simulink model "DC_DC"  (R2021a)
settings: Solver=ode4  StartTime=0.0  StopTime=10.0  FixedStep=10e-6  RelTol=1e-3
libraries: spsSeriesRLCBranchLib x4, spsCurrentMeasurementLib x3, spsVoltageMeasurementLib x3, spsMeanLib x2, spsRMSLib x2, spsDiodeLib x1, spsFirstOrderFilterLib x1, spsIGBTDiodeLib x1, spsPermanentMagnetSynchronousMachineLib x1, simulink x1, spsThreePhaseVIMeasurementLib x1, spsUniversalBridgeLib x1
settings Model: Creator=Sourav Das  LastModifiedBy=Sourav Das

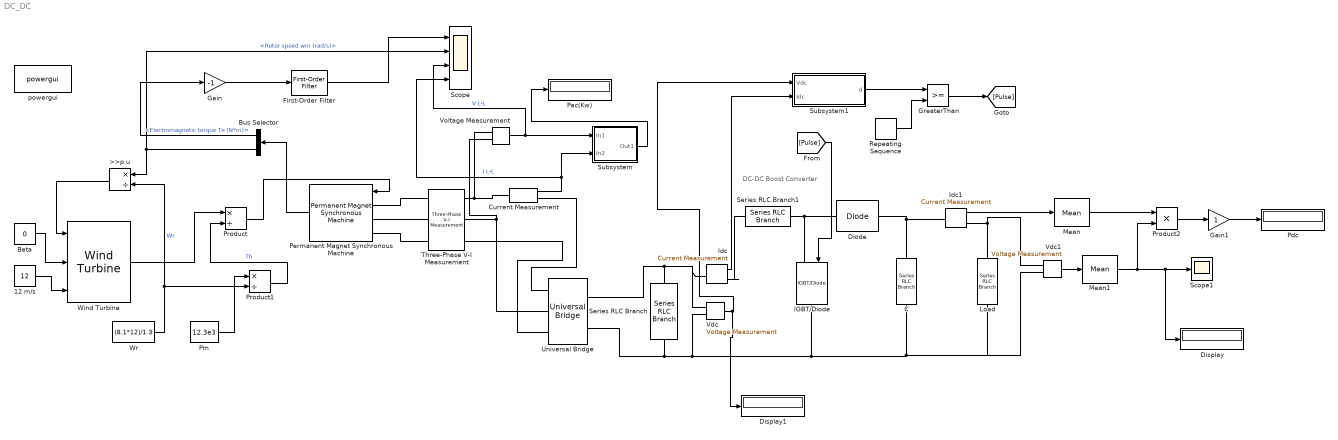
== system DC_DC ==
  note: DC-DC Boost Converter
  12 m/s : Constant  Value=12
  >>p.u : Product  Inputs=*/
  Beta : Constant  Value=0
  Bus Selector : BusSelector  OutputSignals=Electromagnetic torque Te (N*m),Rotor speed wm (rad/s)
  C : spsSeriesRLCBranchLib/Series RLC Branch  LConnTagsString=__new0  RConnTagsString=__new0  BranchType=RC  Resistance=0.005  Inductance=1e-3  SetiL0=off  InitialCurrent=0  Capacitance=6.6094e-04  Setx0=off  InitialVoltage=0  Measurements=None
  Current Measurement : spsCurrentMeasurementLib/Current Measurement  PhasorSimulation=off  OutputType=Complex  PSBequivalent=0
  Diode : spsDiodeLib/Diode  Ron=0.001  Lon=0  Vf=0.8  IC=0  UseSnubber=0  Rs=inf  Cs=inf  Measurements=off
  Display : Display
  Display1 : Display
  First-Order Filter : spsFirstOrderFilterLib/First-Order Filter  FilterType=Lowpass  Tc=10e-3  Ts=50e-6  Initialize=on  Vac_Init=[0, 0, 50]  Vdc_Init=0  PlotResponse=off  FreqRange="[0,  200,  1]"
  Gain : Gain  Gain=-1
  Gain1 : Gain
  GreaterThan : RelationalOperator  OutDataTypeStr=boolean  RndMeth=Simplest
  IGBT/Diode : spsIGBTDiodeLib/IGBT//Diode  Ron=1e-3  Rs=1e5  Cs=inf  Measurements=off
  Idc : spsCurrentMeasurementLib/Current Measurement  PhasorSimulation=off  OutputType=Complex  PSBequivalent=0
  Idc1 : spsCurrentMeasurementLib/Current Measurement  PhasorSimulation=off  OutputType=Complex  PSBequivalent=0
  Load : spsSeriesRLCBranchLib/Series RLC Branch  LConnTagsString=__new0  RConnTagsString=__new0  BranchType=R  Resistance=13.5  Inductance=1e-3  SetiL0=off  InitialCurrent=0  Capacitance=500e-6  Setx0=off  InitialVoltage=0  Measurements=None
  Mean : spsMeanLib/Mean  Freq=50  Vinit=0  Ts=50e-6
  Mean1 : spsMeanLib/Mean  Freq=50  Vinit=0  Ts=50e-6
  Pac(Kw) : Display
  Pdc : Display
  Permanent Magnet Synchronous Machine : spsPermanentMagnetSynchronousMachineLib/Permanent Magnet Synchronous Machine  NbPhases=3  FluxDistribution=Sinusoidal  RotorType=Salient-pole  MechanicalLoad=Torque Tm  PresetModel=No  ShowDetailedParameters=on  MeasurementBus=off  Resistance=0.0485  Inductance=8.5e-3  dqInductances=[0.395e-3,0.395e-3]  La=0.000395  MachineConstant=Flux linkage established by magnets (V.s)  Flux=0.1194  VoltageCst=86.6271  TorqueCst=0.7164  Flat=120  Mechanical=[0.0027 0.0004924 4 0]  PolePairs=4  InitialConditions=[0,0, 0,0]  InitialConditions5ph=[0 0 0 0 0 0]  RefAngle=90 degrees behind phase A axis (modified Park)  IterativeDiscreteModel=Trapezoidal non iterative  TsBlock=-1  TsPowergui=0
  Pm : Constant  Value=12.3e3
  Product : Product  Inputs=*/
  Product1 : Product  Inputs=*/
  Product2 : Product
  Repeating Sequence : simulink/Sources/Repeating Sequence  rep_seq_t=[0 1/20000]  rep_seq_y=[0 0.9]
  Scope : Scope  NumInputPorts=4
  Scope1 : Scope
  Series RLC Branch : spsSeriesRLCBranchLib/Series RLC Branch  LConnTagsString=__new0  RConnTagsString=__new0  BranchType=RC  Resistance=0.005  Inductance=1e-3  SetiL0=off  InitialCurrent=0  Capacitance=500e-6  Setx0=off  InitialVoltage=0  Measurements=None
  Series RLC Branch1 : spsSeriesRLCBranchLib/Series RLC Branch  LConnTagsString=__new0  RConnTagsString=__new0  BranchType=L  Resistance=0.005  Inductance=4.5573e-05  SetiL0=off  InitialCurrent=0  Capacitance=500e-6  Setx0=off  InitialVoltage=0  Measurements=None
  Subsystem : Subsystem
  Subsystem1 : Subsystem
  Three-Phase V-I Measurement : spsThreePhaseVIMeasurementLib/Three-Phase V-I Measurement  VoltageMeasurement=no  SetLabelV=off  LabelV=Vabc  Vpu=off  VpuLL=off  CurrentMeasurement=no  SetLabelI=off  LabelI=Iabc  Ipu=off  Pbase=100e6  Vbase=500e3  OutputType=Complex  PhasorSimulation=off  PSBequivalent=0
  Universal Bridge : spsUniversalBridgeLib/Universal Bridge  Arms=3  SnubberResistance=1e5  SnubberCapacitance=inf  Device=Diodes  Ron=1e-3  Lon=0  ForwardVoltages="[  0  0  ]"  ForwardVoltage=0  GTOparameters=[ 10e-6 , 20e-6 ]  IGBTparameters=[ 1e-6 , 2e-6 ]  Measurements=None  Measurements_2=None  converterType=Rectifier
  Vdc : spsVoltageMeasurementLib/Voltage Measurement  PhasorSimulation=off  OutputType=Complex  PSBequivalent=0
  Vdc1 : spsVoltageMeasurementLib/Voltage Measurement  PhasorSimulation=off  OutputType=Complex  PSBequivalent=0
  Voltage Measurement : spsVoltageMeasurementLib/Voltage Measurement  PhasorSimulation=off  OutputType=Complex  PSBequivalent=0
  Wind Turbine : spsWindTurbineLib/Wind Turbine  Pnom=12.3e6  Pelec_base=12.3e6/0.9  wind_base=12  P_wind_base=0.85  speed_nom=1.2  pitch_angle=0  c1_c6="[0.51763          116          0.4            5           21     0.006795]"  cp_nom=0.48  lambda_nom=8.1
      link override Gain: Gain=-1
      settings: SourceProductBaseCode=PS
  Wr : Constant  Value=(8.1*12)/1.3
  powergui : spspowerguiLib/powergui  Priority=1  SimulationMode=Discrete  SampleTime=20e-6  frequency=60  Iterations=50  frequencyindice=0  Pbase=100e6  ErrMax=1e-4  UnitsV=kV  UnitsW=MW  buscounter=0  FunctionMessages=off  echomessages=off  EnableUseOfTLC=off  CurrentSourceSwitches=off  DisableSnubberDevices=off  DisableRonSwitches=off  DisableVfSwitches=off  DisplayEquations=off  AutomaticDiscreteSolvers=off  SolverType=Tustin/Backward Euler (TBE)  Interpol=off  ExternalGateDelay=off  methode=off  Ts=100  x0status=blocks  SPID=on  SwTol=0  HookPort=off  NonlinearTolerance=1e-4  nMaxIteration=100  ContinueOnMaxIteration=off  RestoreLinks=warning  ResistiveCurrentMeasurement=off  Frange=[0:2:500]  Ylog=off  Xlog=on  ShowGrid=off  save=off  variable=ZData  structure=0  ZoomFFT=off  StartTime=0.0  cycles=1  DisplayStyle=1  fundamental=60  FreqAxis=off  MaxFrequency=1000  frequencyindicesteady=1  RmsSteady=1  display=off
  wires:
  Beta/1 -> Wind Turbine/2
  Wind Turbine/1 -> Product/1
  Pm/1 -> Product1/1
  Wr/1 -> Product1/2, >>p.u/2  "Wr"
  Product1/1 -> Product/2  "Tb"
  Product/1 -> Permanent Magnet Synchronous Machine/1
  Permanent Magnet Synchronous Machine/1 -> Bus Selector/1
  Bus Selector/1 -> Gain/1  "<Electromagnetic torque Te (N*m)>"
  Bus Selector/2 -> Scope/2, >>p.u/1  "<Rotor speed wm (rad/s)>"
  >>p.u/1 -> Wind Turbine/1
  12 m/s/1 -> Wind Turbine/3
  First-Order Filter/1 -> Scope/1
  Gain/1 -> First-Order Filter/1
  Voltage Measurement/1 -> Scope/3, Subsystem/1(In1)  "V L-L"
  Current Measurement/1 -> Scope/4, Subsystem/2(In2)  "I L-L"
  Subsystem/1(Out1) -> Pac(Kw)/1
  Vdc/1 -> Display1/1, Subsystem1/1(Vdc)
  Idc/1 -> Subsystem1/2(Idc)
  Subsystem1/1(d) -> GreaterThan/1
  Repeating Sequence/1 -> GreaterThan/2
  GreaterThan/1 -> [Pulse]
  Idc1/1 -> Mean/1
  Vdc1/1 -> Mean1/1
  Mean/1 -> Product2/1
  Mean1/1 -> Display/1, Scope1/1, Product2/2
  Product2/1 -> Gain1/1
  Gain1/1 -> Pdc/1
  [Pulse] -> IGBT/Diode/1
  connections:
  Permanent Magnet Synchronous Machine/LConn1 -- Three-Phase V-I Measurement/LConn1
  Permanent Magnet Synchronous Machine/LConn2 -- Three-Phase V-I Measurement/LConn2
  Permanent Magnet Synchronous Machine/LConn3 -- Three-Phase V-I Measurement/LConn3
  Three-Phase V-I Measurement/RConn2 -- Voltage Measurement/LConn2 -- Universal Bridge/LConn2
  Three-Phase V-I Measurement/RConn3 -- Universal Bridge/LConn3
  Three-Phase V-I Measurement/RConn1 -- Voltage Measurement/LConn1 -- Current Measurement/LConn1
  Current Measurement/RConn1 -- Universal Bridge/LConn1
  Universal Bridge/RConn1 -- Idc/LConn1 -- Vdc/LConn1 -- Series RLC Branch/LConn1
  Universal Bridge/RConn2 -- Vdc1/LConn2 -- Load/RConn1 -- C/RConn1 -- IGBT/Diode/RConn1 -- Vdc/LConn2 -- Series RLC Branch/RConn1
  Idc/RConn1 -- Series RLC Branch1/RConn1
  IGBT/Diode/LConn1 -- Diode/LConn1 -- Series RLC Branch1/LConn1
  Diode/RConn1 -- Idc1/LConn1 -- C/LConn1
  Load/LConn1 -- Vdc1/LConn1 -- Idc1/RConn1

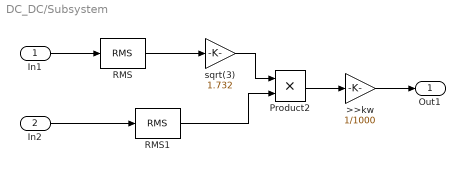
== system DC_DC/Subsystem ==
  In1 : Inport
  In2 : Inport  Port=2
  >>kw : Gain  Gain=1/1000
  Product2 : Product
  RMS : spsRMSLib/RMS  TrueRMS=on  Freq=50  RMSInit=120  Ts=50e-6
  RMS1 : spsRMSLib/RMS  TrueRMS=on  Freq=50  RMSInit=120  Ts=50e-6
  sqrt(3) : Gain  Gain=1.732
  Out1 : Outport
  wires:
  RMS1/1 -> Product2/2
  In1/1 -> RMS/1
  RMS/1 -> sqrt(3)/1
  sqrt(3)/1 -> Product2/1
  In2/1 -> RMS1/1
  Product2/1 -> >>kw/1
  >>kw/1 -> Out1/1

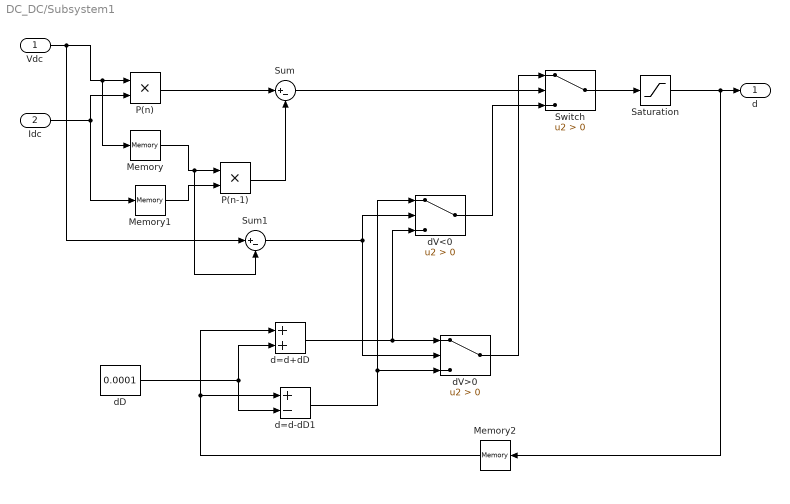
== system DC_DC/Subsystem1 ==
  Vdc : Inport
  Idc : Inport  Port=2
  Memory : Memory
  Memory1 : Memory
  Memory2 : Memory
  P(n) : Product
  P(n-1) : Product
  Saturation : Saturate  UpperLimit=inf
  Sum : Sum  Inputs=|+-
  Sum1 : Sum  Inputs=|+-
  Switch : Switch  Criteria=u2 > Threshold
  d=d+dD : Sum
  d=d-dD1 : Sum  Inputs=+-
  dD : Constant  Value=0.0001
  dV<0 : Switch  Criteria=u2 > Threshold
  dV>0 : Switch  Criteria=u2 > Threshold
  d : Outport
  wires:
  Vdc/1 -> Sum1/1, Memory/1, P(n)/1
  Idc/1 -> P(n)/2, Memory1/1
  Memory/1 -> Sum1/2, P(n-1)/1
  Memory1/1 -> P(n-1)/2
  P(n)/1 -> Sum/1
  P(n-1)/1 -> Sum/2
  Sum/1 -> Switch/2
  Switch/1 -> Saturation/1
  Memory2/1 -> d=d-dD1/1, d=d+dD/1
  dD/1 -> d=d-dD1/2, d=d+dD/2
  Sum1/1 -> dV>0/2, dV<0/2
  d=d-dD1/1 -> dV>0/3, dV<0/1
  d=d+dD/1 -> dV>0/1, dV<0/3
  dV>0/1 -> Switch/1
  dV<0/1 -> Switch/3
  Saturation/1 -> d/1, Memory2/1
